simulink model "MovingAverage"  (R2024a)
settings: Solver=FixedStepDiscrete  StartTime=0.0  StopTime=inf  FixedStep=0.01  RelTol=1e-3  EnableMultiTasking=on
settings Model: Creator=USER  LastModifiedBy=USER
settings SolverCC: PositivePriorityOrder=on
settings OptimizationCC: EnhancedBackFolding=on  PassReuseOutputArgsAs=Individual arguments  ZeroExternalMemoryAtStartup=off  ZeroInternalMemoryAtStartup=off  MaxStackSize=200000  OptimizeBlockOrder=speed  DifferentSizesBufferReuse=on  OptimizationCustomize=off  EfficientTunableParamExpr=on
settings DebuggingCC: ParameterTunabilityLossMsg=error
settings HardwareCC: ProdBitPerPointer=32  ProdBitPerSizeT=32  ProdBitPerPtrDiffT=32  ProdLargestAtomicInteger=Long  ProdLargestAtomicFloat=Double  ProdWordSize=32  ProdLongLongMode=on  ProdHWDeviceType=ARM Compatible->ARM Cortex-A (32-bit)  UseEmbeddedCoderFeatures=off
settings RTWCC: Description=Embedded Coder  SystemTargetFile=ert.tlc  HardwareBoard=Raspberry Pi  TLCOptions="-aInlineSetEventsForThisBaseRateFcn=TLC_FALSE -aSuppressMultiTaskScheduler=TLC_FALSE  -aRateBasedStepFcn=0"  TemplateMakefile=ert_default_tmf  RTWVerbose=off  Toolchain=GNU GCC Embedded Linux  BuildConfiguration=Faster Runs
settings CodeAppCC: ForceParamTrailComments=on  IgnoreCustomStorageClasses=off  OperatorAnnotations=on  SimulinkDataObjDesc=on  SFDataObjDesc=on  InsertBlockDesc=on
settings ERTTargetCC: SupportNonInlinedSFcns=on  SupportVariableSizeSignals=on  ExtModeTransport=2  ExtModeStaticAlloc=on  ExtModeMexFile=ext_xcp  ExtModeIntrfLevel=Level2 - Open
settings ConfigComp: CovBoundaryAbsTol=1.0e-5

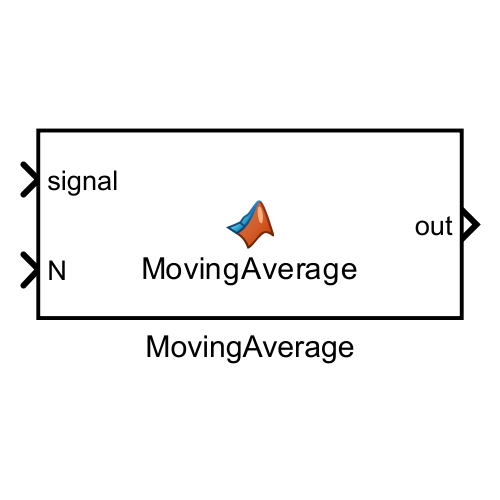
[thumbnail: Simulink's stored preview of the top-level diagram]
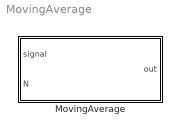
== system MovingAverage ==
  MovingAverage : MATLAB Function  TreatAsAtomicUnit=on

== matlab function MovingAverage/MovingAverage ==
  data: signal input; out output; N input
function out = MovingAverage(signal, N)

    signal = double(signal);

    persistent buf idx count sumval

    if isempty(buf)
        MAX_N = 200;
        buf    = zeros(MAX_N, 1, 'double');
        idx    = int32(1);
        count  = int32(0);
        sumval = 0.0;
    end

    MAX_N = length(buf);
    Ni = int32(N);
    if Ni < 1
        Ni = int32(1);
    elseif Ni > MAX_N
        Ni = int32(MAX_N);
    end

    old = buf(idx);
    sumval = sumval - old + signal;
    buf(idx) = signal;

    idx = idx + 1;
    if idx > Ni
        idx = int32(1);
    end

    if count < Ni
        count = count + 1;
    end

    out = sumval / double(count);
end
